simulink model "Flow_Meter"  (R2017b)
settings: Solver=FixedStepAuto  StartTime=0.0  StopTime=1  RelTol=1e-3
libraries: dspsigops x1
settings Model: Creator=Vishnu  LastModifiedBy=Vishnu
settings OptimizationCC: DefaultParameterBehavior=Inlined  UseDivisionForNetSlopeComputation=on  UseFloatMulNetSlope=on  InlineInvariantSignals=on  EnhancedBackFolding=on  BooleansAsBitfields=on  PassReuseOutputArgsAs=Individual arguments  StateBitsets=on  DataBitsets=on  ZeroExternalMemoryAtStartup=off  ZeroInternalMemoryAtStartup=off  NoFixptDivByZeroProtection=on  EfficientFloat2IntCast=on  LifeSpan=1
settings DebuggingCC: ParameterTunabilityLossMsg=error
settings SFSimCC: MATLABDynamicMemAlloc=off
settings RTWCC: SystemTargetFile=ert.tlc  TemplateMakefile=ert_default_tmf  GenerateReport=on  IncludeHyperlinkInReport=on  LaunchReport=on  GenerateTraceInfo=on  GenerateTraceReport=on  GenerateTraceReportSl=on  GenerateTraceReportSf=on  GenerateTraceReportEml=on  GenerateCodeMetricsReport=on
settings CodeAppCC: ForceParamTrailComments=on  IgnoreCustomStorageClasses=off  OperatorAnnotations=on  SimulinkDataObjDesc=on  SFDataObjDesc=on  CustomSymbolStrGlobalVar=rt$N$M  CustomSymbolStrType=$N$M  CustomSymbolStrFcn=$N$M$F  CustomSymbolStrMacro=$N$M  InsertBlockDesc=on
settings ERTTargetCC: TargetLangStandard=C99 (ISO)  GenerateSampleERTMain=on  IncludeMdlTerminateFcn=off  CombineSignalStateStructs=on  SupportComplex=off  SupportContinuousTime=on  SupportNonInlinedSFcns=on  InlinedParameterPlacement=NonHierarchical  ERTCustomFileTemplate=example_file_process.tlc  ERTFilePackagingFormat=CompactWithDataFile

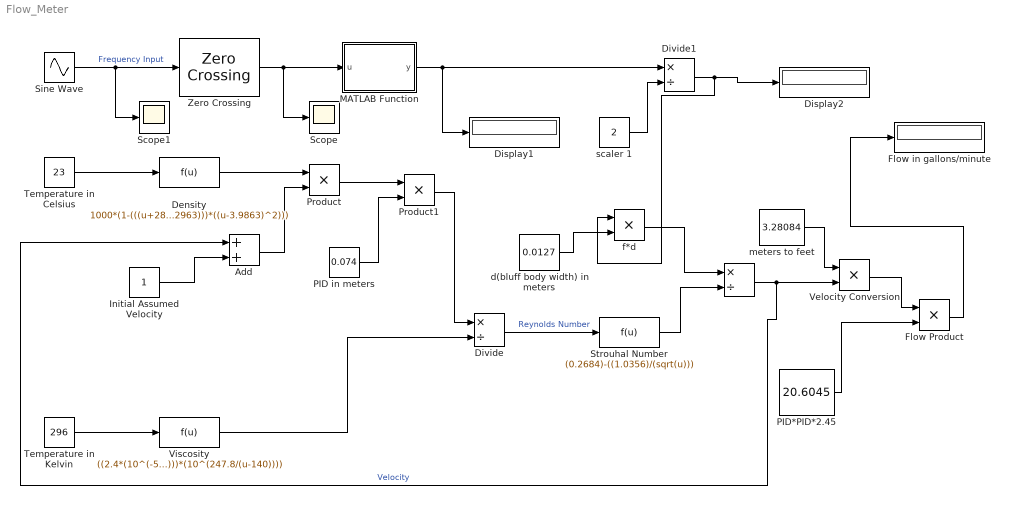
== system Flow_Meter ==
  " " : Product  Inputs=*/
  Add : Sum
  "Density " : Fcn  Expr=1000*(1-(((u+288.9414)/((508929.2)*(u+68.12963)))*((u-3.9863)^2)))
  Display1 : Display
  Display2 : Display
  Divide : Product  Inputs=*/
  Divide1 : Product  Inputs=*/
  Flow Product : Product
  "Flow in gallons/minute " : Display
  Initial Assumed Velocity : Constant
  MATLAB Function : MATLAB Function  TreatAsAtomicUnit=on
  PID in meters : Constant  Value=0.074
  PID*PID*2.45 : Constant  Value=20.6045
  Product : Product
  Product1 : Product
  Scope : Scope
  Scope1 : Scope
  "Sine Wave " : Sin  Amplitude=5  Frequency=2*pi*2000  Samples=5  SampleTime=0  VectorParams1D=off
  Strouhal Number : Fcn  Expr=(0.2684)-((1.0356)/(sqrt(u)))
  Temperature in Celsius : Constant  Value=23
  "Temperature in Kelvin " : Constant  Value=296
  Velocity Conversion : Product
  Viscosity : Fcn  Expr=((2.4*(10^(-5)))*(10^(247.8/(u-140))))
  Zero Crossing : dspsigops/Zero Crossing
      settings: SourceProductName=DSP System Toolbox  SourceProductBaseCode=DS
  d(bluff body width) in meters : Constant  Value=0.0127
  f*d : Product
  "meters to feet " : Constant  Value=3.28084
  scaler 1 : Constant  Value=2
  wires:
  "Temperature in Kelvin "/1 -> Viscosity/1
  Temperature in Celsius/1 -> "Density "/1
  "Density "/1 -> Product/1
  Product/1 -> Product1/1
  PID in meters/1 -> Product1/2
  Product1/1 -> Divide/1
  Viscosity/1 -> Divide/2
  Divide/1 -> Strouhal Number/1  "Reynolds Number"
  d(bluff body width) in meters/1 -> f*d/2
  f*d/1 -> " "/1
  Strouhal Number/1 -> " "/2
  " "/1 -> Add/1, Velocity Conversion/2  "Velocity"
  PID*PID*2.45/1 -> Flow Product/2
  Flow Product/1 -> "Flow in gallons/minute "/1
  "Sine Wave "/1 -> Scope1/1, Zero Crossing/1  "Frequency Input"
  Zero Crossing/1 -> Scope/1, MATLAB Function/1(u)
  MATLAB Function/1(y) -> Divide1/1, Display1/1
  scaler 1/1 -> Divide1/2
  Divide1/1 -> f*d/1, Display2/1
  "meters to feet "/1 -> Velocity Conversion/1
  Velocity Conversion/1 -> Flow Product/1
  Initial Assumed Velocity/1 -> Add/2
  Add/1 -> Product/2

== matlab function Flow_Meter/MATLAB Function ==
  data: u input; y output
function y = fcn(u)
persistent count1
if isempty(count1)
    count1=1
end
if u > 0
    count1=count1+1
end
y = count1;
